simulink model "SistemaCAS_v13"  (R2014a)
settings: Solver=ode3  StartTime=0.0  StopTime=1  FixedStep=0.001  RelTol=1e-3
libraries: commchan3 x1
settings Model: Creator=andre  LastModifiedBy=andre
settings DebuggingCC: SolverPrmCheckMsg=none

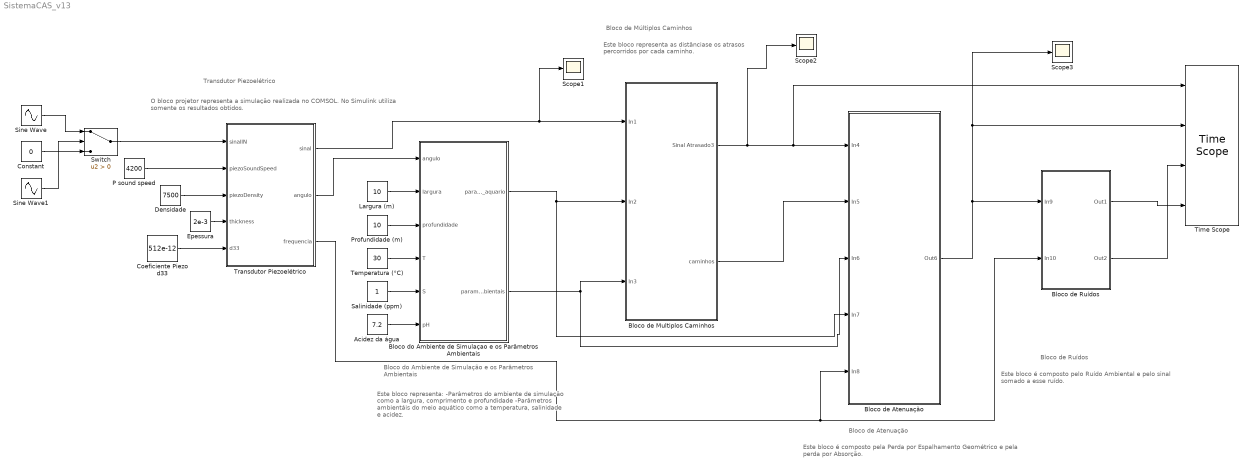
== system SistemaCAS_v13 ==
  note: O bloco projetor representa a simulação realizada no COMSOL. No Simulink utiliza somente os resultados obtidos.
  note: Transdutor Piezoelétrico
  note: Este bloco representa:
      | -Parâmetros do ambiente de simulação como a largura, comprimento e profundidade
      | -Parâmetros ambientáis do meio aquático como a temperatura, salinidade e acidez.
  note: Bloco do Ambiente de Simulação e os Parâmetros Ambientais
  note: Este bloco representa as distânciase os atrasos percorridos por cada caminho.
  note: Bloco de Múltiplos Caminhos
  note: Este bloco é composto pela Perda por Espalhamento Geométrico e pela perda por Absorção.
  note: Bloco de Atenuação
  note: Este bloco é composto pelo Ruído Ambiental e pelo sinal somado a esse ruído.
  note: Bloco de Ruídos
  Acidez da água : Constant  Value=7.2
  Bloco de Atenuação : Subsystem
  Bloco de Multiplos Caminhos : Subsystem
  Bloco de Ruídos : Subsystem
  Bloco do Ambiente de Simulaçao e os Parâmetros Ambientais : MATLAB Function  TreatAsAtomicUnit=on
  Coeficiente Piezo d33 : Constant  Value=512e-12
  Constant : Constant  Value=0
  Densidade : Constant  Value=7500
  Epessura : Constant  Value=2e-3
  Largura (m) : Constant  Value=10
  P sound speed : Constant  Value=4200
  Profundidade (m) : Constant  Value=10
  Salinidade (ppm) : Constant
  Scope1 : Scope
      settings: YMin=-10  YMax=10
  Scope2 : Scope
      settings: YMin=-10  YMax=10
  Scope3 : Scope
      settings: YMin=-10  YMax=10  SaveName=ScopeData2
  Sine Wave : Sin  Amplitude=10  Frequency=100  Phase=0.15  SampleTime=0
  Sine Wave1 : Sin  SampleTime=0
  Switch : Switch  Criteria=u2 > Threshold
  Temperatura (°C) : Constant  Value=30
  Time Scope : TimeScope  NumInputPorts=4  DefaultConfigurationName=spbscopes.TimeScopeBlockCfg
  Transdutor Piezoelétrico : MATLAB Function  TreatAsAtomicUnit=on
  wires:
  Sine Wave/1 -> Switch/1
  Sine Wave1/1 -> Switch/2
  Constant/1 -> Switch/3
  Largura (m)/1 -> Bloco do Ambiente de Simulaçao e os Parâmetros Ambientais/2(largura)
  Profundidade (m)/1 -> Bloco do Ambiente de Simulaçao e os Parâmetros Ambientais/3(profundidade)
  Coeficiente Piezo d33/1 -> Transdutor Piezoelétrico/5(d33)
  P sound speed/1 -> Transdutor Piezoelétrico/2(piezoSoundSpeed)
  Densidade/1 -> Transdutor Piezoelétrico/3(piezoDensity)
  Epessura/1 -> Transdutor Piezoelétrico/4(thickness)
  Transdutor Piezoelétrico/2(angulo) -> Bloco do Ambiente de Simulaçao e os Parâmetros Ambientais/1(angulo)
  Transdutor Piezoelétrico/1(sinal) -> Scope1/1, Bloco de Multiplos Caminhos/1(In1)
  Bloco do Ambiente de Simulaçao e os Parâmetros Ambientais/1(parametros_aquario) -> Bloco de Atenuação/4(In7), Bloco de Multiplos Caminhos/2(In2)
  Bloco do Ambiente de Simulaçao e os Parâmetros Ambientais/2(parametros_ambientais) -> Bloco de Multiplos Caminhos/3(In3), Bloco de Atenuação/3(In6)
  Switch/1 -> Transdutor Piezoelétrico/1(sinalIN)
  Transdutor Piezoelétrico/3(frequencia) -> Bloco de Atenuação/5(In8), Bloco de Ruídos/2(In10)
  Temperatura (°C)/1 -> Bloco do Ambiente de Simulaçao e os Parâmetros Ambientais/4(T)
  Salinidade (ppm)/1 -> Bloco do Ambiente de Simulaçao e os Parâmetros Ambientais/5(S)
  Acidez da água/1 -> Bloco do Ambiente de Simulaçao e os Parâmetros Ambientais/6(pH)
  Bloco de Multiplos Caminhos/1(Sinal Atrasado3) -> Scope2/1, Time Scope/1, Bloco de Atenuação/1(In4)
  Bloco de Ruídos/1(Out1) -> Time Scope/4
  Bloco de Multiplos Caminhos/2(caminhos) -> Bloco de Atenuação/2(In5)
  Bloco de Atenuação/1(Out6) -> Scope3/1, Time Scope/2, Bloco de Ruídos/1(In9)
  Bloco de Ruídos/2(Out2) -> Time Scope/3

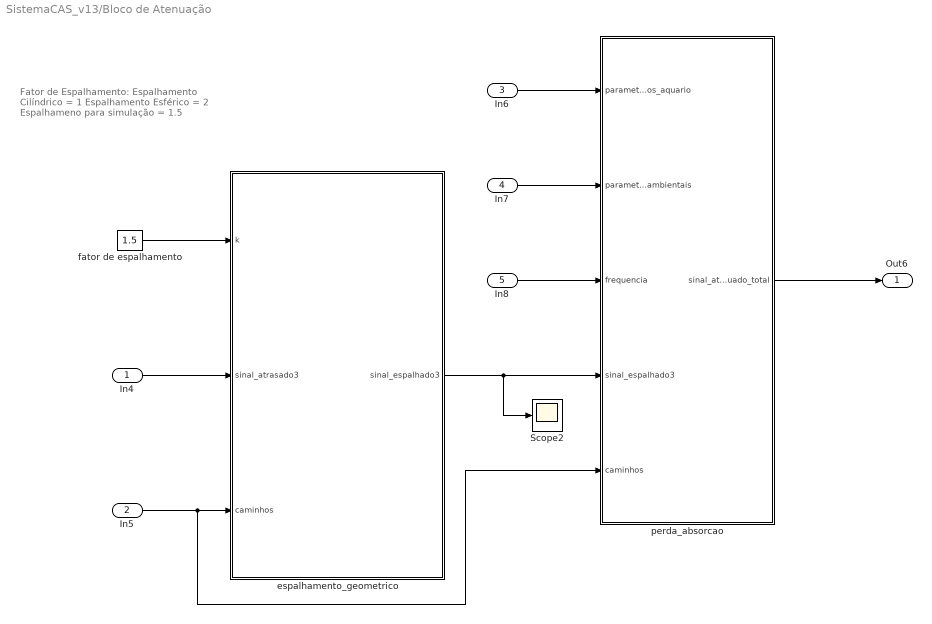
== system SistemaCAS_v13/Bloco de Atenuação ==
  note: Fator de Espalhamento:
      | Espalhamento Cilíndrico = 1
      | Espalhamento Esférico = 2
      | Espalhameno para simulação = 1.5
  In4 : Inport
  In5 : Inport  Port=2
  In6 : Inport  Port=3
  In7 : Inport  Port=4
  In8 : Inport  Port=5
  Scope2 : Scope
      settings: YMin=-10  YMax=10  SaveName=ScopeData3
  espalhamento_geometrico : MATLAB Function  TreatAsAtomicUnit=on
  fator de espalhamento : Constant  Value=1.5
  perda_absorcao : MATLAB Function  TreatAsAtomicUnit=on
  Out6 : Outport
  wires:
  fator de espalhamento/1 -> espalhamento_geometrico/1(k)
  espalhamento_geometrico/1(sinal_espalhado3) -> Scope2/1, perda_absorcao/4(sinal_espalhado3)
  perda_absorcao/1(sinal_atenuado_total) -> Out6/1
  In4/1 -> espalhamento_geometrico/2(sinal_atrasado3)
  In5/1 -> perda_absorcao/5(caminhos), espalhamento_geometrico/3(caminhos)
  In6/1 -> perda_absorcao/1(parametros_aquario)
  In7/1 -> perda_absorcao/2(parametros_ambientais)
  In8/1 -> perda_absorcao/3(frequencia)

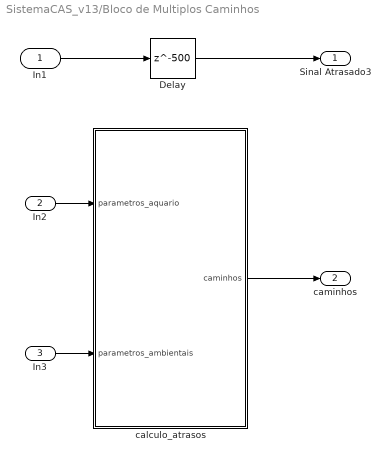
== system SistemaCAS_v13/Bloco de Multiplos Caminhos ==
  In1 : Inport
  In2 : Inport  Port=2
  In3 : Inport  Port=3
  Delay : Delay  DelayLength=500  InitialCondition=0
  calculo_atrasos : MATLAB Function  TreatAsAtomicUnit=on
  Sinal Atrasado3 : Outport
  caminhos : Outport  Port=2
  wires:
  In2/1 -> calculo_atrasos/1(parametros_aquario)
  In3/1 -> calculo_atrasos/2(parametros_ambientais)
  In1/1 -> Delay/1
  Delay/1 -> Sinal Atrasado3/1
  calculo_atrasos/1(caminhos) -> caminhos/1

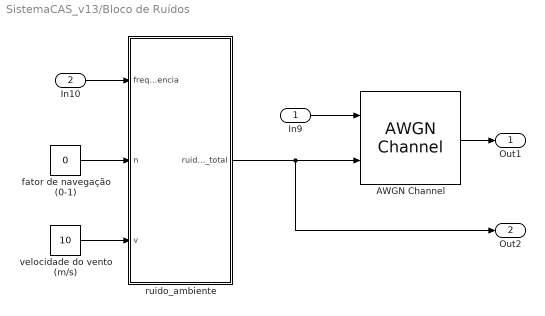
== system SistemaCAS_v13/Bloco de Ruídos ==
  In9 : Inport
  In10 : Inport  Port=2
  AWGN Channel : commchan3/AWGN Channel  InputProcessing=Columns as channels (frame based)  seed=5  noiseMode=Variance from port  EbNodB=10  EsNodB=10  SNRdB=10  bitsPerSym=1  Ps=1  Tsym=1  variance=1
  fator de navegação (0-1) : Constant  Value=0
  ruido_ambiente : MATLAB Function  TreatAsAtomicUnit=on
  velocidade do vento (m/s) : Constant  Value=10
  Out1 : Outport
  Out2 : Outport  Port=2
  wires:
  In10/1 -> ruido_ambiente/1(frequencia)
  ruido_ambiente/1(ruido_total) -> Out2/1, AWGN Channel/2
  AWGN Channel/1 -> Out1/1
  In9/1 -> AWGN Channel/1
  fator de navegação (0-1)/1 -> ruido_ambiente/2(n)
  velocidade do vento (m/s)/1 -> ruido_ambiente/3(v)

== matlab function SistemaCAS_v13/Bloco do Ambiente de Simulaçao e os Parâmetros Ambientais ==
  data: angulo input; largura input; profundidade input; parametros_aquario output; parametros_ambientais output; T input; S input; pH input
function [parametros_aquario,parametros_ambientais] = ambiente_simulado(angulo,largura,profundidade,T,S,pH)
% consideraçoes para os parâmetros do aquário
% 1. emissor e receptor estão alinhados ( largura(x) e profundidade(z)
% iguais, só muda o comprimento (y)
% 2. o comprimento do aquario (L) é ideal para acontecer uma reflexão completa
% com o angulo de diretividade (que é o maior angulo possível do lóbulo 
% principal utilizando o transdutor piezoeletrico escolhido)
% 3. para facilitar os cálculos de do comprimento ideal, utilizamos largura
% igual profundidade (D = W)

% considerações sobre a simulação
% 1. serão considerados somente os caminhos do angulo de diretividade e o
% caminho direto (5 caminhos: um direto, dois que refletem nas laterais, e
% dois que refletem na superfície e o fundo
% 2. a reflexão será considerada reflexão completa com um eco (sem perdas 
% de energia ou refraçao)

%-------------------------------------------------------------------------
%Parâmetros do Aquário definidos anteriormente
%-------------------------------------------------------------------------
W = largura;                  % largura (eixo x)
D = profundidade;             % profundidade do aquário (eixo z) 
L = W/sin(angulo/2);      % comprimento do aquário calculado utilizando o angulo de diretividade (eixo y)
% l(éle) é a distancia ideal para acontecer uma reflexão completa
parametros_aquario = [W,L,D];


%-------------------------------------------------------------------------
% Valores dos parâmetros do meio subaquático 
%-------------------------------------------------------------------------
%T = 30;                 % Temperatura (°C)
%S = 1;                  % Salinidade (ppt)
%pH = 7.2;               % acidêz da água - pH (potencial hidrogeniônico)
parametros_ambientais = [T, S, pH];

== matlab function SistemaCAS_v13/Bloco de Multiplos Caminhos/calculo_atrasos ==
  data: parametros_aquario input; parametros_ambientais input; caminhos output
function caminhos  = calculo_atrasos(parametros_aquario,parametros_ambientais)
%Definir as distâncias de cada caminho do multipath;
%Definir a profundidade media para cada caminho do multipath;
%Equação para Velocidade do som na água; 
%Atrasar o sinal de cada caminho do multipath;

%-------------------------------------------------------------------------
% Parametros do aquário e do ambiente que serao utilizados no código 
%-------------------------------------------------------------------------

W = parametros_aquario(1);      %W é a largura do aquário
L = parametros_aquario(2);      %L é comprimento do aquário
D = parametros_aquario(3);      %D é a profundidade do aquário

T = parametros_ambientais(1);   %T é a temperatura da água;
S = parametros_ambientais(2);   %S é a salinidade da água;
pH = parametros_ambientais(3);  %pH é acidez da água;

%-------------------------------------------------------------------------
% Definindo as distâncias em metros de cada caminho do multipath entre o 
% emissor e o receptor
%-------------------------------------------------------------------------
% caminho(1) = caminho refletido na superfície
% caminho(2) = caminho refletido na lateral de trás
% caminho(3) = caminho direto
% caminho(4) = caminho refletido na lateral da frente
% caminho(5) = caminho refletido no fundo
%-------------------------------------------------------------------------


%caminhos(1) = sqrt(D^2 + L^2);
%caminhos(2) = sqrt(W^2 + L^2);  
caminhos = L                %L é comprimento do aquário
%caminhos(4) = caminhos(2);
%caminhos(5) = sqrt(D^2 + L^2);

%-------------------------------------------------------------------------
%Definindo a profundidade média(Dm) para cada caminho, considerando que os
%transdutores estão localizados na metade do aquário e alinhados entre si.
%-------------------------------------------------------------------------


%Dm(1) = mean([D/2,0]);
%Dm(2) = D/2;
Dm = D/2
%Dm(4) = D/2;
%Dm(5) = mean([D,D/2]);

%-------------------------------------------------------------------------
%Equação que define a Velocidade do som na água em (m/s)
%-------------------------------------------------------------------------


C = 1448.96 + 4.591*T - 5.304*(10^(-2))*(T^(2))...
    + 2.374*(10^(-4))*(T^(3)) + 1.340*(S-35) + 1.630*(10^(-2))*Dm...
    + 1.675*(10^(-7))*(Dm^(2)) - 1.025*(10^(-2))*T*(S-35)...
    - 7.139*(10^(-13))*T*(Dm^(3))

%-------------------------------------------------------------------------
% Definindo os atrasos em segundos para cada caminho do multipath.
% O atraso é descoberto através da divisão da distância em metros 
% pela velocidade do som na agua em metros/segundos.
%-------------------------------------------------------------------------

%atraso1 = caminhos(1)/C(1);
%atraso2 = caminhos(2)/C(2);
%atraso3 = caminhos/C % caminho direto não tem atraso
%atraso4 = caminhos(4)/C(4);
%atraso5 = caminhos(5)/C(5);

== matlab function SistemaCAS_v13/Bloco de Atenuação/perda_absorcao ==
  data: parametros_aquario input; parametros_ambientais input; frequencia input; sinal_espalhado3 input; caminhos input; sinal_atenuado_total output
function sinal_atenuado_total = perda_absorcao(parametros_aquario,parametros_ambientais,...
    frequencia,sinal_espalhado3,caminhos)

% Parâmetros Ambientais
T = parametros_ambientais(1);
S = parametros_ambientais(2);
pH = parametros_ambientais(3);

%Profundidade
D = parametros_aquario(3);

%Valores dos parâmetros Ácido Bórico(f1) e Sulfato de Magnésio(f2)
f1 = 0.78 * sqrt(S/35) * (exp(T/26))
f2 = 42 * (exp(T/17))

%Absorption Coefficient
a = ((0.106 * (f1 * frequencia^2) * exp((pH - 8)/0.56)) / (f1^2 + frequencia^2)) +...
    ((0.52 * (1 + (T/43)) * (S/45) * (f2 * frequencia^2) *...
    exp(-(D/6))) / (f2^2 + frequencia^2)) + (0.00049 * (frequencia^2) * (exp(-(T/27 + D/17))))

% Perda_absorção = 10log(a)*r (dB)
% a é o coeficiente de absorção que depende da frequência. 
% Para um dado valor de frequência, a absorção varia linerarmente com a 
% faixa r em quilometros.

caminhos
%atenuação em db
%atenuacao1 = 10*log(a)*caminhos(1);
%atenuacao2 = 10*log(a)*caminhos(2);
atenuacao3 = 10*log(a)*caminhos
%atenuacao4 = 10*log(a)*caminhos(4);
%atenuacao5 = 10*log(a)*caminhos(5);
atenuacaomag = db2mag(atenuacao3)
sinal_espalhado3
% sinal atenuado em magnitude
%sinal_atenuado1 = db2mag(atenuacao1).*sinal_espalhado1;
%sinal_atenuado2 = db2mag(atenuacao2).*sinal_espalhado2;
sinal_atenuado3 = db2mag(atenuacao3).*sinal_espalhado3
%sinal_atenuado4 = db2mag(atenuacao4).*sinal_espalhado4;
%sinal_atenuado5 = db2mag(atenuacao5).*sinal_espalhado5;

sinal_atenuado_total = sinal_atenuado3

== matlab function SistemaCAS_v13/Bloco de Atenuação/espalhamento_geometrico ==
  data: k input; sinal_atrasado3 input; sinal_espalhado3 output; caminhos input
function sinal_espalhado3  = espalhamento_geometrico(k,sinal_atrasado3,caminhos)
% a perda por espalhamento geométrico é calculado a partir da equação 
%perda_espalhamento = k * 10log(r); equação da dissertação
%k = fator de espalhamento
%caminhos = distância em metros
%perda_espalhamento_caminho(2) = 37,38 (para k=1)
%perda_espalhamento_caminho(2) = 22,46 (para k=1,5)
%perda_espalhamento_caminho(2) = 31,45 (para k=2)

%espalhamento1 = k * 10*log(caminhos(1));
%espalhamento2 = k * 10*log(caminhos(2));
espalhamento3 = k * 10*log(caminhos)
%espalhamento4 = k * 10*log(caminhos(4));
%espalhamento5 = k * 10*log(caminhos(5));

% sinal espalhado

espmag = db2mag(espalhamento3)
sinal_atrasado3

%sinal_espalhado1 = db2mag(espalhamento1).*sinal_atrasado1;
%sinal_espalhado2 = db2mag(espalhamento2).*sinal_atrasado2;
sinal_espalhado3 = db2mag(espalhamento3).*sinal_atrasado3
%sinal_espalhado4 = db2mag(espalhamento4).*sinal_atrasado4;
%sinal_espalhado5 = db2mag(espalhamento5).*sinal_atrasado5;

== matlab function SistemaCAS_v13/Transdutor Piezoelétrico ==
  data: sinalIN input; sinal output; piezoSoundSpeed input; piezoDensity input; thickness input; d33 input; angulo output; frequencia output
function [sinal,angulo,frequencia] = projetor(sinalIN, piezoSoundSpeed, piezoDensity, thickness, d33)
%-------------------------------------------------------------------------
% Sinal 
%-------------------------------------------------------------------------
sinal=sinalIN

%-------------------------------------------------------------------------
% Ângulo de diretividade do transdutor calculado no COMSOL (rad)
%(ex.: 60º = pi/3 rad)
%-------------------------------------------------------------------------
angulo = pi/4;            % 45°

%-------------------------------------------------------------------------
% Frequência do Sinal (kHz)
%-------------------------------------------------------------------------
frequencia = 16120;

== matlab function SistemaCAS_v13/Bloco de Ruídos/ruido_ambiente ==
  data: ruido_total output; frequencia input; n input; v input
function ruido_total  = ruido_ambiente(frequencia,n,v)
% frequência (kHz); 
f = frequencia;
% n - fator de navegaçao(entre 0 - 1);
% v - velocidade do vento (m/s); 

%Equaçao do Ruído de Turbulência
Nt = (10^((17-30*log10(f))/10));

%Equação do Ruído de Navegações
Ns = (10^((40+(20*(n-0.5))+(26*log10(f))-(60*log10(f+0.03)))/10));

%Equação do Ruído das Ondas
Nw = (10^((50+(7.5*(v^(1/2)))+(20*log10(f))-(40*log10(f+0.4)))/10));

%Equação do Ruído Térmico
Nth = (10^((-15+20*log10(f))/10));

%Ruído Total somado em dB
ruido_total = Nt + Ns + Nw + Nth;
